simulink model "QCS_Sim"  (Simulink 9.1)
settings: Solver=ode45  StartTime=0.0  StopTime=4  RelTol=1e-3  EnableMultiTasking=on
libraries: cstblocks x8
settings Model: SuppressorTable=22 serialization::archive 11 0 6 0 0 0 0 0  Creator=Mokrane  LastModifiedBy=Mokrane
settings DataIOCC: LimitDataPoints=on  SignalLoggingSaveFormat=ModelDataLogs  SignalLoggingName=sigsOut
settings OptimizationCC: LifeSpan=auto
settings DebuggingCC: SaveWithParameterizedLinksMsg=none  SignalResolutionControl=TryResolveAllWithWarning  MultiTaskDSMMsg=warning  MultiTaskCondExecSysMsg=none  SFUnexpectedBacktrackingDiag=error  SFNoUnconditionalDefaultTransitionDiag=error  SFExecutionAtInitializationDiag=warning
settings HardwareCC: TargetUnknown=on
settings CodeAppCC: StateflowObjectComments=off

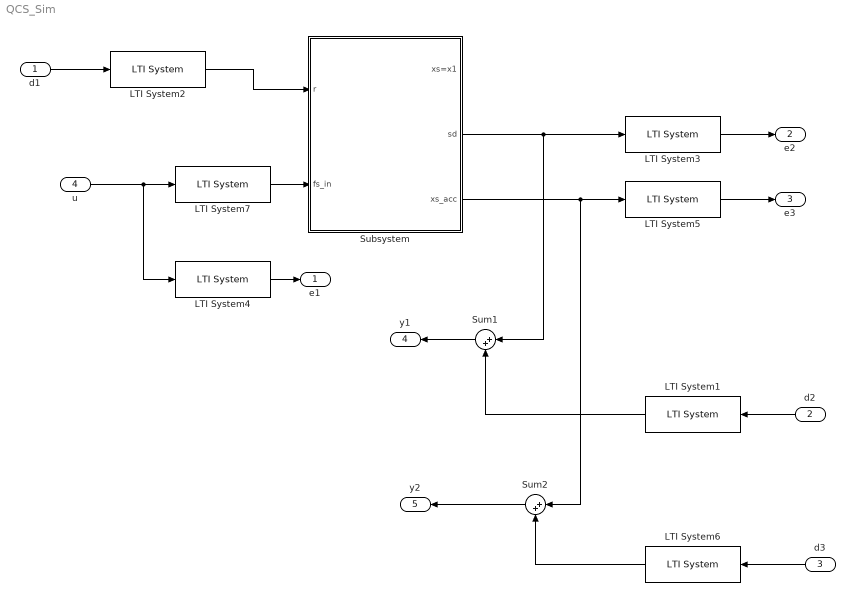
== system QCS_Sim ==
  d1 : Inport
  d2 : Inport  Port=2
  d3 : Inport  Port=3
  u : Inport  Port=4
  LTI System1 : cstblocks/LTI System  sys=Wd2  IC=[]
  LTI System2 : cstblocks/LTI System  sys=Wroad  IC=[]
  LTI System3 : cstblocks/LTI System  sys=Wsd  IC=[]
  LTI System4 : cstblocks/LTI System  sys=Wact  IC=[]
  LTI System5 : cstblocks/LTI System  sys=Wab  IC=[]
  LTI System6 : cstblocks/LTI System  sys=Wd3  IC=[]
  LTI System7 : cstblocks/LTI System  sys=Act  IC=[]
  Subsystem : Subsystem
  Sum1 : Sum  Inputs=|++  SaturateOnIntegerOverflow=on
  Sum2 : Sum  Inputs=|++  SaturateOnIntegerOverflow=on
  e1 : Outport
  e2 : Outport  Port=2
  e3 : Outport  Port=3
  y1 : Outport  Port=4
  y2 : Outport  Port=5
  wires:
  d1/1 -> LTI System2/1
  LTI System2/1 -> Subsystem/1(r)
  LTI System4/1 -> e1/1
  Subsystem/2(sd) -> LTI System3/1, Sum1/1
  LTI System3/1 -> e2/1
  Subsystem/3(xs_acc) -> Sum2/1, LTI System5/1
  LTI System5/1 -> e3/1
  d2/1 -> LTI System1/1
  d3/1 -> LTI System6/1
  LTI System1/1 -> Sum1/2
  Sum1/1 -> y1/1
  LTI System6/1 -> Sum2/2
  Sum2/1 -> y2/1
  u/1 -> LTI System7/1, LTI System4/1
  LTI System7/1 -> Subsystem/2(fs_in)

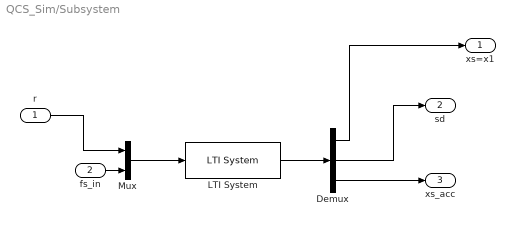
== system QCS_Sim/Subsystem ==
  r : Inport
  fs_in : Inport  Port=2
  Demux : Demux  Outputs=3
  LTI System : cstblocks/LTI System  sys=qcar  IC=[]
  Mux : Mux  Inputs=2
  xs=x1 : Outport
  sd : Outport  Port=2
  xs_acc : Outport  Port=3
  wires:
  Demux/2 -> sd/1
  Demux/3 -> xs_acc/1
  Demux/1 -> xs=x1/1
  r/1 -> Mux/1
  fs_in/1 -> Mux/2
  Mux/1 -> LTI System/1
  LTI System/1 -> Demux/1
